simulink model "Actuator_Model"  (R2018b)
settings: Solver=VariableStepAuto  StartTime=0.0  StopTime=200  RelTol=1e-3
values from neighbouring files (symbols this model uses):
  J_r = 0.0004    [Lab1.m]    (also in Micro_Sat_Open_Loop.m)
  Tc_max = 0.05    [Lab1.m]    (also in Micro_Sat_Open_Loop.m)
undefined symbols (not defined in the file or in its folder): sigbuilder_block
settings Model: Creator=EKOCULU  LastModifiedBy=EKOCULU

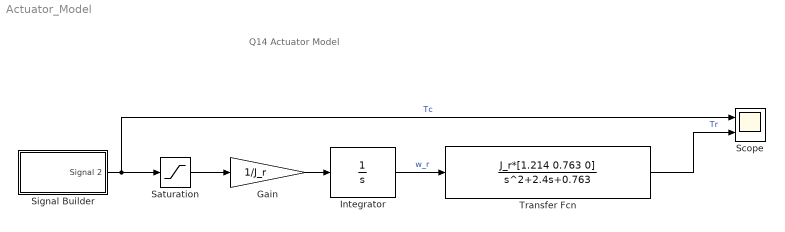
== system Actuator_Model ==
  note: Q14 Actuator Model
  Gain : Gain  Gain=1/J_r
  Integrator : Integrator  LimitOutput=on  UpperSaturationLimit=2800*pi/30  LowerSaturationLimit=-2800*pi/30
  Saturation : Saturate  UpperLimit=Tc_max  LowerLimit=-Tc_max
  Scope : Scope  NumInputPorts=2
  Signal Builder : Subsystem  Tag=STV Subsys  LoadFcn=sigbuilder_block('load');  StartFcn=sigbuilder_block('start');  StopFcn=sigbuilder_block('stop');  ClipboardFcn=sigbuilder_block('clipboard');  mask(Sigbuilder block){tuvar=[0:10]}
      mask help: Simulink:masks:SigbuilderBlock_MD
      mask init:
      | if ~strcmp(get_param(bdroot(gcbh),'SimulationStatus'),'stopped') tuvar = sigbuilder_block('maskInit'); end
      settings: CopyFcn=sigbuilder_block('copy');  DeleteFcn=sigbuilder_block('delete');  ModelCloseFcn=sigbuilder_block('modelClose');  PreSaveFcn=sigbuilder_block('preSave');  PauseFcn=sigbuilder_block('pause');  ContinueFcn=sigbuilder_block('continue');  NameChangeFcn=sigbuilder_block('namechange');  OpenFcn=sigbuilder_block('open',[106.5 72.75 1122.75 636 ]);  CloseFcn=sigbuilder_block('close');
      mask Display: plot(0, 0, 100, 100,[2, 2, 32, 32, 2], [68, 8, 8, 68, 68],[32, 2], [38, 38], [32, 19, 2],[53, 60, 44], [32, 17, 17, 2],[16, 16, 31, 31]);txt = getActiveGroup(gcbh);text(2, 100, txt,'verticalAlignment', 'top');
  Transfer Fcn : TransferFcn  Numerator=J_r*[1.214 0.763 0]  Denominator=[1 2.4 0.763]
  wires:
  Transfer Fcn/1 -> Scope/2  "Tr"
  Signal Builder/1(Signal 2) -> Scope/1, Saturation/1  "Tc"
  Integrator/1 -> Transfer Fcn/1  "w_r"
  Gain/1 -> Integrator/1
  Saturation/1 -> Gain/1

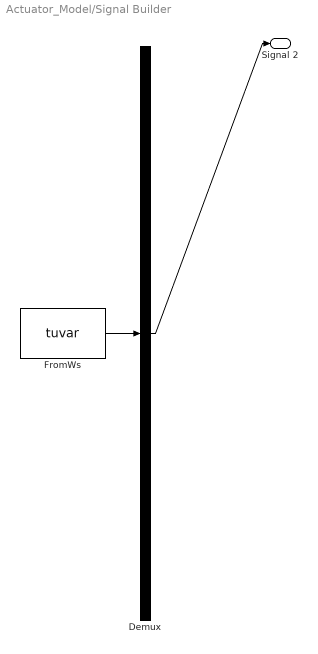
== system Actuator_Model/Signal Builder ==
  Demux : Demux  Tag=STV Demux  Outputs=1
  FromWs : FromWorkspace  Tag=STV FromWs  VariableName=tuvar  SampleTime=0
      SigBuilderData=|
      | common.afterFinalStr = 'Extrapolate'
      | common.sampleTime = 0
      | dataSet.timeRange = [0 200]
      | dataSet.name = 'Group 1'
      | sbobj.Groups.Name = 'Group 1'
      | sbobj.Groups.Signals.Name = 'Signal 2'
      | sbobj.Groups.Signals.XData = [0 20 20 80 80 139.8 139.8 140 140 200]
      | sbobj.Groups.Signals.YData = [0 0 0.003 0.003 -0.003 -0.003 0 0 1e-05 1e-05]
      | sbobj.Groups.TimeRange = [0 200]
  Signal 2 : Outport  Tag=STV Outport
  wires:
  FromWs/1 -> Demux/1
  Demux/1 -> Signal 2/1
